simulink model "kinematic_step_mpc"  (R2015b)
settings: Solver=FixedStepAuto  StartTime=0.0  StopTime=20  FixedStep=0.01  RelTol=1e-3
values from neighbouring files (symbols this model uses):
  Lf = 1    [KINEMATIC_MOTION_PLANNER.m]    (also in KINEMATIC_MOTION_PLANNER2.m; KINEMATIC_STEP_MPC.m; KINEMATIC_VEHICLE_CONTROL.m; KINEMATIC_VEHICLE_SIM.m)
  Lr = 1    [KINEMATIC_MOTION_PLANNER.m]    (also in KINEMATIC_MOTION_PLANNER2.m; KINEMATIC_STEP_MPC.m; KINEMATIC_VEHICLE_CONTROL.m; KINEMATIC_VEHICLE_SIM.m)
  Psi0 = 0    [KINEMATIC_MOTION_PLANNER.m]    (also in KINEMATIC_MOTION_PLANNER2.m; KINEMATIC_STEP_MPC.m; KINEMATIC_VEHICLE_CONTROL.m; KINEMATIC_VEHICLE_SIM.m)
  V = 1    [KINEMATIC_MOTION_PLANNER.m]    (also in KINEMATIC_MOTION_PLANNER2.m; KINEMATIC_STEP_MPC.m; KINEMATIC_VEHICLE_CONTROL.m; KINEMATIC_VEHICLE_SIM.m = 5)
  X0 = 0    [KINEMATIC_MOTION_PLANNER.m]    (also in KINEMATIC_MOTION_PLANNER2.m; KINEMATIC_STEP_MPC.m; KINEMATIC_VEHICLE_CONTROL.m; KINEMATIC_VEHICLE_SIM.m)
  Y0 = 0    [KINEMATIC_MOTION_PLANNER.m]    (also in KINEMATIC_MOTION_PLANNER2.m; KINEMATIC_STEP_MPC.m; KINEMATIC_VEHICLE_CONTROL.m; KINEMATIC_VEHICLE_SIM.m)
settings Model: Creator=gebruiker  LastModifiedBy=gebruiker

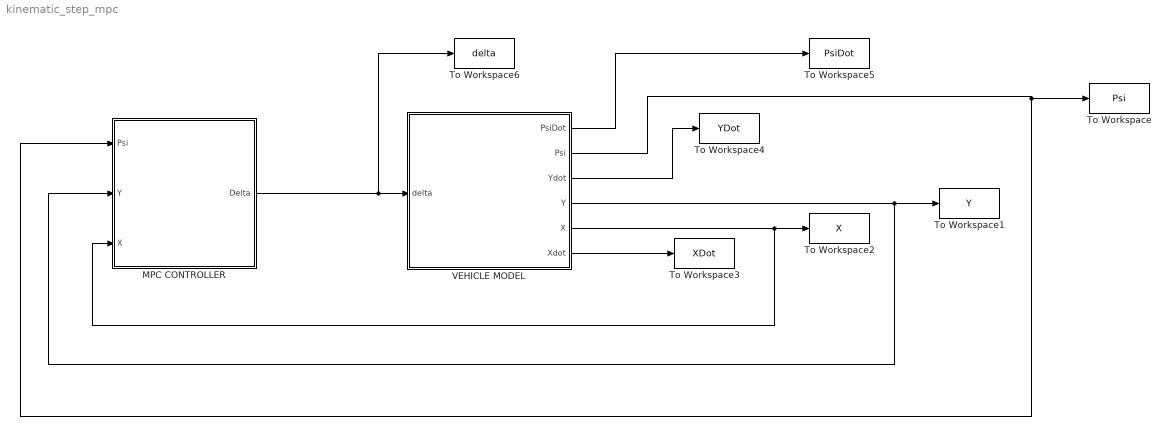
== system kinematic_step_mpc ==
  MPC CONTROLLER : Subsystem
  To Workspace : ToWorkspace  VariableName=Psi  SaveFormat=Structure With Time  SampleTime=-1
  To Workspace1 : ToWorkspace  VariableName=Y  SaveFormat=Structure With Time  SampleTime=-1
  To Workspace2 : ToWorkspace  VariableName=X  SaveFormat=Structure With Time  SampleTime=-1
  To Workspace3 : ToWorkspace  VariableName=XDot  SaveFormat=Structure With Time  SampleTime=-1
  To Workspace4 : ToWorkspace  VariableName=YDot  SaveFormat=Structure With Time  SampleTime=-1
  To Workspace5 : ToWorkspace  VariableName=PsiDot  SaveFormat=Structure With Time  SampleTime=-1
  To Workspace6 : ToWorkspace  VariableName=delta  SaveFormat=Structure With Time  SampleTime=-1
  VEHICLE MODEL : Subsystem
  wires:
  VEHICLE MODEL/1(PsiDot) -> To Workspace5/1
  VEHICLE MODEL/2(Psi) -> To Workspace/1, MPC CONTROLLER/1(Psi)
  VEHICLE MODEL/3(Ydot) -> To Workspace4/1
  VEHICLE MODEL/4(Y) -> MPC CONTROLLER/2(Y), To Workspace1/1
  VEHICLE MODEL/5(X) -> To Workspace2/1, MPC CONTROLLER/3(X)
  VEHICLE MODEL/6(Xdot) -> To Workspace3/1
  MPC CONTROLLER/1(Delta) -> To Workspace6/1, VEHICLE MODEL/1("delta ")

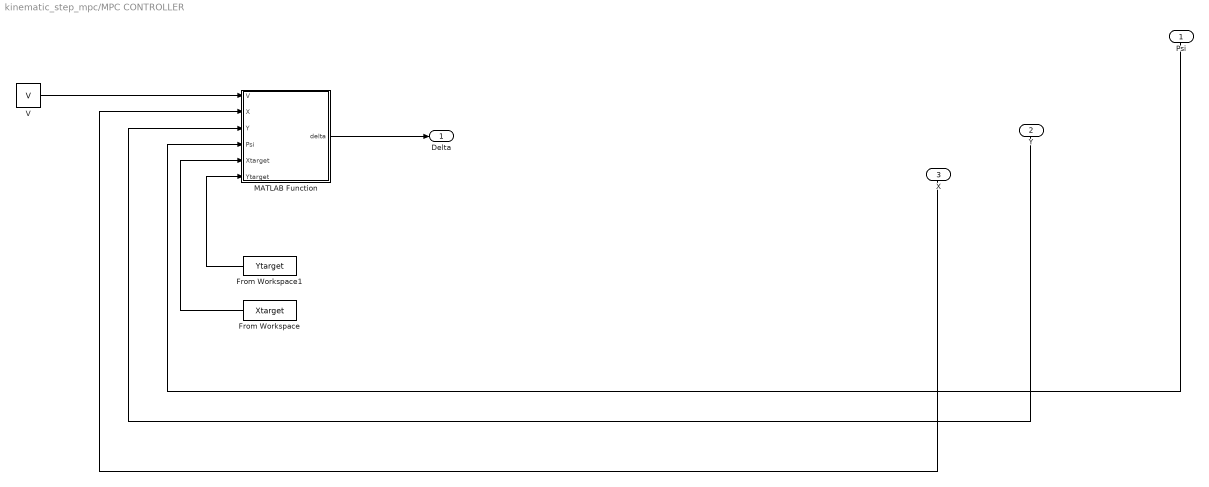
== system kinematic_step_mpc/MPC CONTROLLER ==
  Psi : Inport
  Y : Inport  Port=2
  X : Inport  Port=3
  From Workspace : FromWorkspace  VariableName=Xtarget  SampleTime=0
  From Workspace1 : FromWorkspace  VariableName=Ytarget  SampleTime=0
  MATLAB Function : MATLAB Function  TreatAsAtomicUnit=on
  "V " : Constant  Value=V
  Delta : Outport
  wires:
  "V "/1 -> MATLAB Function/1(V)
  Y/1 -> MATLAB Function/3(Y)
  Psi/1 -> MATLAB Function/4(Psi)
  X/1 -> MATLAB Function/2(X)
  MATLAB Function/1(delta) -> Delta/1
  From Workspace/1 -> MATLAB Function/5(Xtarget)
  From Workspace1/1 -> MATLAB Function/6(Ytarget)

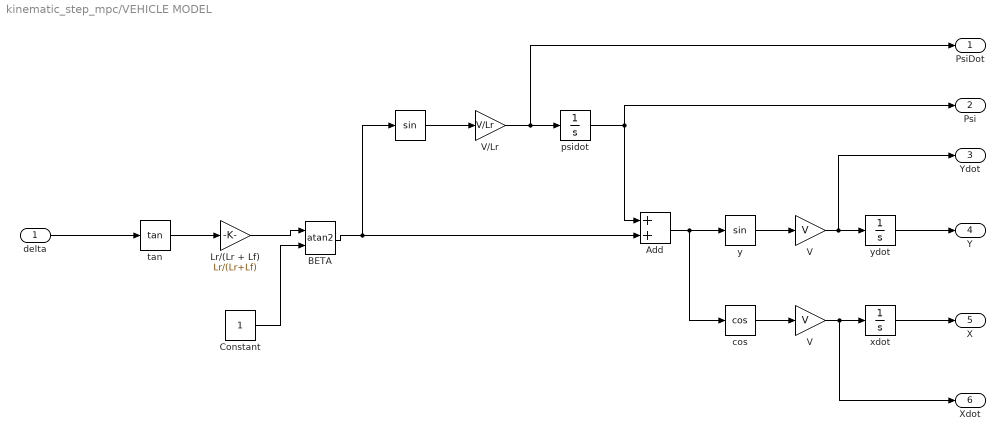
== system kinematic_step_mpc/VEHICLE MODEL ==
  "delta " : Inport
  " " : Trigonometry
  Add : Sum
  BETA : Trigonometry  Operator=atan2
  Constant : Constant
  Lr/(Lr + Lf) : Gain  Gain=Lr/(Lr+Lf)
  V : Gain  Gain=V
  "V " : Gain  Gain=V
  V/Lr : Gain  Gain=V/Lr
  cos : Trigonometry  Operator=cos
  psidot : Integrator  InitialCondition=Psi0
  "tan " : Trigonometry  Operator=tan
  xdot : Integrator  InitialCondition=X0
  y : Trigonometry
  ydot : Integrator  InitialCondition=Y0
  PsiDot : Outport
  Psi : Outport  Port=2
  Ydot : Outport  Port=3
  Y : Outport  Port=4
  X : Outport  Port=5
  Xdot : Outport  Port=6
  wires:
  V/1 -> Ydot/1, ydot/1
  Lr/(Lr + Lf)/1 -> BETA/1
  BETA/1 -> Add/2, " "/1
  "V "/1 -> Xdot/1, xdot/1
  Add/1 -> cos/1, y/1
  xdot/1 -> X/1
  ydot/1 -> Y/1
  psidot/1 -> Psi/1, Add/1
  "delta "/1 -> "tan "/1
  V/Lr/1 -> PsiDot/1, psidot/1
  y/1 -> V/1
  " "/1 -> V/Lr/1
  "tan "/1 -> Lr/(Lr + Lf)/1
  cos/1 -> "V "/1
  Constant/1 -> BETA/2

== matlab function kinematic_step_mpc/MPC CONTROLLER/MATLAB Function ==
  data: V input; delta output; X input; Y input; Psi input; Xtarget input; Ytarget input
function delta = fcn(V,X,Y,Psi,Xtarget,Ytarget)
%#codegen
% 
dt = 0.1;
R = [cos(Psi), -sin(Psi);sin(Psi),cos(Psi)];
Lmin = 1000;
delta_best = 0;
for delta = linspace(-pi/6,pi/6,21)
    dx = V*dt;
    dy = 2*V*delta*dt;
    drot = R*[dx;dy];
    Xfin = X + drot(1);
    Yfin = Y + drot(2);
    L = sqrt((Xtarget - Xfin)^2+(Ytarget - Yfin)^2);
    if L < Lmin
        Lmin = L;
        delta_best = delta;
    end
end
delta = delta_best;
end
